simulink model "gm_HDLHeaderFull_vs"  (R2024a)
settings: Solver=FixedStepDiscrete  StartTime=0.0  StopTime=stopTime  RelTol=1e-3
values from neighbouring files (symbols this model uses):
  fs = 1    [testHeaderFull.m]
undefined symbols (not defined in the file or in its folder): clk, clk_enable, headerBitsPerFec, headerBitsPerOFDMSymbol, reset_x
libraries: hdlsllib x30, whdlutilities x6, simulink x5, dspsrcs4 x5, commhdlcrc x1, whdledac x1, vivadosimlib x1, HDL_ieee_8021513 x1
settings Model: Creator=cotti  LastModifiedBy=cotti
settings OptimizationCC: BlockReduction=off  ConditionallyExecuteInputs=off  DefaultParameterBehavior=Inlined  InheritOutputTypeSmallerThanSingle=on
settings DebuggingCC: AlgebraicLoopMsg=error  ArtificialAlgebraicLoopMsg=error  InheritedTsInSrcMsg=none  SingleTaskRateTransMsg=error  UnconnectedInputMsg=warning  UnconnectedOutputMsg=warning  UnconnectedLineMsg=warning
settings HardwareCC: ProdBitPerPointer=32  ProdBitPerSizeT=32  ProdBitPerPtrDiffT=32  ProdLargestAtomicFloat=None  ProdIntDivRoundTo=Undefined  ProdEndianess=Unspecified  ProdWordSize=32  ProdHWDeviceType=ASIC/FPGA->ASIC/FPGA  TargetBitPerLong=64  TargetBitPerPointer=64  TargetBitPerSizeT=64  TargetBitPerPtrDiffT=64  TargetLongLongMode=on  TargetIntDivRoundTo=Zero  TargetEndianess=LittleEndian  TargetWordSize=64  TargetHWDeviceType=Custom Processor->MATLAB Host Computer  ProdEqTarget=off

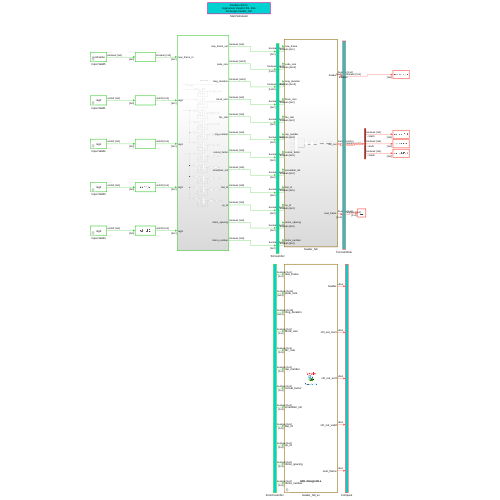
[thumbnail: Simulink's stored preview of the top-level diagram]
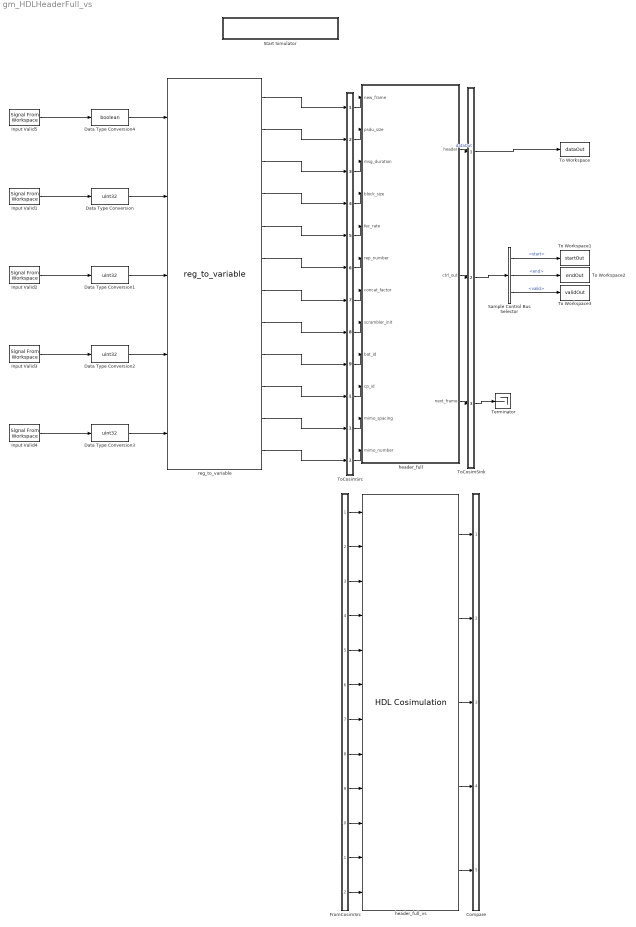
== system gm_HDLHeaderFull_vs ==
  Compare : Subsystem
      mask Display: disp('')
  Data Type Conversion{,1..3} (4 alike) : DataTypeConversion  OutDataTypeStr=uint32  SaturateOnIntegerOverflow=off  RndMeth=Floor
  Data Type Conversion4 : DataTypeConversion  OutDataTypeStr=boolean  SaturateOnIntegerOverflow=off  RndMeth=Floor
  FromCosimSrc : Subsystem
      mask Display: disp('')
  Input Valid1 : dspsrcs4/Signal From Workspace  X=reg0  Ts=1/fs  nsamps=1  OutputAfterFinalValue=Setting to zero  ignoreOrWarnInputAndFrameLengths=off  OutputFrames=off
  Input Valid2 : dspsrcs4/Signal From Workspace  X=reg1  Ts=1/fs  nsamps=1  OutputAfterFinalValue=Setting to zero  ignoreOrWarnInputAndFrameLengths=off  OutputFrames=off
  Input Valid3 : dspsrcs4/Signal From Workspace  X=reg2  Ts=1/fs  nsamps=1  OutputAfterFinalValue=Setting to zero  ignoreOrWarnInputAndFrameLengths=off  OutputFrames=off
  Input Valid4 : dspsrcs4/Signal From Workspace  X=reg3  Ts=1/fs  nsamps=1  OutputAfterFinalValue=Setting to zero  ignoreOrWarnInputAndFrameLengths=off  OutputFrames=off
  Input Valid5 : dspsrcs4/Signal From Workspace  X=newFrame  Ts=1/fs  nsamps=1  OutputAfterFinalValue=Setting to zero  ignoreOrWarnInputAndFrameLengths=off  OutputFrames=off
  Sample Control Bus Selector : whdlutilities/Sample Control Bus Selector  OutputSignals=start,end,valid
  Start Simulator : Subsystem
      settings: OpenFcn=|
      | cosimDirName = pwd;
      | cd 'hdl_prj_header_full/hdlsrc/HDLHeaderFull';
      | [s,r] = system('vivado -mode batch -source gm_HDLHeaderFull_vs.tcl','-echo');
      | cd (cosimDirName);
      | clear cosimDirName;
      | if s
      |    error('Failed to create Vivado HDL design DLL using script gm_HDLHeaderFull_vs.tcl.');
      | end
      mask Display: disp('Double-click to\nregenerate Vivado HDL DLL\nfor design header_full')
  Terminator : Terminator
  To Workspace : ToWorkspace  VariableName=dataOut  SampleTime=1/(8*fs)
      settings: Save2DSignal=2-D array (concatenate along first dimension)
  To Workspace1 : ToWorkspace  VariableName=startOut  SampleTime=1/(8*fs)
      settings: Save2DSignal=2-D array (concatenate along first dimension)
  To Workspace2 : ToWorkspace  VariableName=endOut  SampleTime=1/(8*fs)
      settings: Save2DSignal=2-D array (concatenate along first dimension)
  To Workspace3 : ToWorkspace  VariableName=validOut  SampleTime=1/(8*fs)
      settings: Save2DSignal=2-D array (concatenate along first dimension)
  ToCosimSink : Subsystem
      mask Display: disp('')
  ToCosimSrc : Subsystem
      mask Display: disp('')
  header_full : Subsystem
  header_full_vs : vivadosimlib/HDL Cosimulation  PortPaths=/header_full/new_frame;/header_full/psdu_size;/header_full/msg_duration;/header_full/block_size;/header_full/fec_rate;/header_full/rep_number;/header_full/concat_factor;/header_full/scrambler_init;/header_full/bat_id;/header_full/cp_id;/header_full/mimo_spacing;/header_full/mimo_number;/header_full/header;/header_full/ctrl_out_start;/header_full/ctrl_out_end;/header_full/ctrl_out_valid;/header_full/next_frame  PortModes=[1 1 1 1 1 1 1 1 1 1 1 1 2 2 2 2 2 ]  PortTimes=[-1 -1 -1 -1 -1 -1 -1 -1 -1 -1 -1 -1 0.125 0.125 0.125 0.125 0.125 ]  PortSigns=[-1 -1 -1 -1 -1 -1 -1 -1 -1 -1 -1 -1 0 0 0 0 0 ]  PortFracLengths=[0,0,0,0,0,0,0,0,0,0,0,0,0,0,0,0,0]  PortWordLengths=[-1,-1,-1,-1,-1,-1,-1,-1,-1,-1,-1,-1,1,1,1,1,1]  PortHDLWordSizes=[1,1,1,1,1,1,1,1,1,1,1,1,1,1,1,1,1]  CommLocal=on  CommSharedMemory=on  CommPortNumber=4449  CommShowInfo=on  ClockPaths=clk;clk_enable;reset_x;  ClockModes=[2 4 3]  ClockTimes=[1e-08 3.7e-08 2.7e-08]  TclPostSimCommand="puts \"done\""  TimingMode=ns  TimingScaleFactor=80  idxCellArray={'UNUSED_VAR'}  CosimBypass=Full Simulation  AllowDirectFeedthrough=on  ProductName=EDA Simulator Link VS  RunAutoTimescale=off  HdlClocks=0  PreRunTime=40  PreRunTimeUnit=ns
  reg_to_variable : HDL_ieee_8021513/reg_to_variable  SystemSampleTime=-1  VariantActivationTime=update diagram  AllowFlexibleInterface=on  Latency=0  AutoFrameSizeCalculation=off
      settings: SourceProductName=HDL IEEE 8021513
  wires:
  Sample Control Bus Selector/2 -> To Workspace2/1  "<end>"
  Sample Control Bus Selector/3 -> To Workspace3/1  "<valid>"
  Sample Control Bus Selector/1 -> To Workspace1/1  "<start>"
  Data Type Conversion/1 -> reg_to_variable/2
  Data Type Conversion1/1 -> reg_to_variable/3
  Data Type Conversion2/1 -> reg_to_variable/4
  Data Type Conversion3/1 -> reg_to_variable/5
  Data Type Conversion4/1 -> reg_to_variable/1
  Input Valid4/1 -> Data Type Conversion3/1
  Input Valid3/1 -> Data Type Conversion2/1
  Input Valid2/1 -> Data Type Conversion1/1
  Input Valid1/1 -> Data Type Conversion/1
  Input Valid5/1 -> Data Type Conversion4/1
  ToCosimSrc/1(out1) -> header_full/1(new_frame)
  ToCosimSrc/2(out2) -> header_full/2(psdu_size)
  ToCosimSrc/3(out3) -> header_full/3(msg_duration)
  ToCosimSrc/4(out4) -> header_full/4(block_size)
  ToCosimSrc/5(out5) -> header_full/5(fec_rate)
  ToCosimSrc/6(out6) -> header_full/6(rep_number)
  ToCosimSrc/7(out7) -> header_full/7(concat_factor)
  ToCosimSrc/8(out8) -> header_full/8(scrambler_init)
  ToCosimSrc/9(out9) -> header_full/9(bat_id)
  ToCosimSrc/10(out10) -> header_full/10(cp_id)
  ToCosimSrc/11(out11) -> header_full/11(mimo_spacing)
  ToCosimSrc/12(out12) -> header_full/12(mimo_number)
  header_full/1(header) -> ToCosimSink/1(in1)  "dataOut"
  header_full/2(ctrl_out) -> ToCosimSink/2(in2)
  header_full/3(next_frame) -> ToCosimSink/3(in3)
  reg_to_variable/1 -> ToCosimSrc/1(in1)
  reg_to_variable/2 -> ToCosimSrc/2(in2)
  reg_to_variable/3 -> ToCosimSrc/3(in3)
  reg_to_variable/4 -> ToCosimSrc/4(in4)
  reg_to_variable/5 -> ToCosimSrc/5(in5)
  reg_to_variable/6 -> ToCosimSrc/6(in6)
  reg_to_variable/7 -> ToCosimSrc/7(in7)
  reg_to_variable/8 -> ToCosimSrc/8(in8)
  reg_to_variable/9 -> ToCosimSrc/9(in9)
  reg_to_variable/10 -> ToCosimSrc/10(in10)
  reg_to_variable/11 -> ToCosimSrc/11(in11)
  reg_to_variable/12 -> ToCosimSrc/12(in12)
  ToCosimSink/1(out1) -> To Workspace/1
  ToCosimSink/2(out2) -> Sample Control Bus Selector/1
  ToCosimSink/3(out3) -> Terminator/1
  FromCosimSrc/1(out1) -> header_full_vs/1
  FromCosimSrc/2(out2) -> header_full_vs/2
  FromCosimSrc/3(out3) -> header_full_vs/3
  FromCosimSrc/4(out4) -> header_full_vs/4
  FromCosimSrc/5(out5) -> header_full_vs/5
  FromCosimSrc/6(out6) -> header_full_vs/6
  FromCosimSrc/7(out7) -> header_full_vs/7
  FromCosimSrc/8(out8) -> header_full_vs/8
  FromCosimSrc/9(out9) -> header_full_vs/9
  FromCosimSrc/10(out10) -> header_full_vs/10
  FromCosimSrc/11(out11) -> header_full_vs/11
  FromCosimSrc/12(out12) -> header_full_vs/12
  header_full_vs/1 -> Compare/1(in1)
  header_full_vs/2 -> Compare/2(in2)
  header_full_vs/3 -> Compare/3(in3)
  header_full_vs/4 -> Compare/4(in4)
  header_full_vs/5 -> Compare/5(in5)

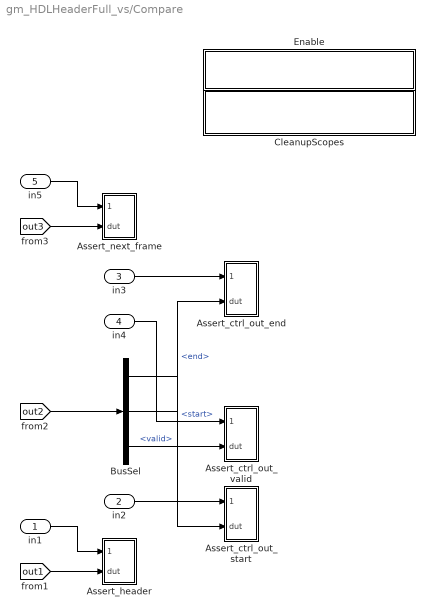
== system gm_HDLHeaderFull_vs/Compare ==
  in1 : Inport
  in2 : Inport  Port=2
  in3 : Inport  Port=3
  in4 : Inport  Port=4
  in5 : Inport  Port=5
  Assert_ctrl_out_end : Subsystem
      settings: LibrarySourceBlock=hdlmdlgenlib/AssertEq
  Assert_ctrl_out_start : Subsystem
      settings: LibrarySourceBlock=hdlmdlgenlib/AssertEq
  Assert_ctrl_out_valid : Subsystem
      settings: LibrarySourceBlock=hdlmdlgenlib/AssertEq
  Assert_header : Subsystem
      settings: LibrarySourceBlock=hdlmdlgenlib/AssertEq
  Assert_next_frame : Subsystem
      settings: LibrarySourceBlock=hdlmdlgenlib/AssertEq
  BusSel : BusSelector  OutputSignals=start,end,valid
  CleanupScopes : Subsystem
      settings: OpenFcn=|
      | blkName = gcb; %self block
      | idx = regexp(blkName, '/CleanupScopes$', 'once');
      | blkParent = blkName(1:idx-1);
      | blks=find_system(blkParent, 'LookUnderMasks', 'all','blocktype', 'Scope');
      | for itr = 1:length(blks)
      | 	 hScopeCfg = get_param(blks{itr},'ScopeConfiguration');
      | 	 hScopeCfg.Visible = ~ hScopeCfg.Visible;
      | end
      | drawnow;
      mask Display: fprintf(message('hdlcoder:cosim:vnl_dblclick').getString());
  Enable : Subsystem
      settings: OpenFcn=|
      | blkName = gcb;
      | idx = regexp(blkName, '/Enable$', 'once');
      | blkParent = blkName(1:idx-1);
      | blks=find_system(blkParent, 'LookUnderMasks', 'all','blocktype', 'Assertion');
      | e = get_param(blks{1}, 'Enabled');
      | if strcmp(e, 'on'), f= 'off';, else, f = 'on';, end
      | for ii=1:length(blks), set_param(blks{ii}, 'Enabled', f);, end
      | set_param(gcb, 'MaskDisplay',['fprintf(message(''hdlcoder:cosim:vnl_dblclick_assertions'',','''',upper(e),'''',').getString())']);
      mask Display: fprintf(message('hdlcoder:cosim:vnl_dblclick_assertions','OFF').getString());
  wires:
  in2/1 -> Assert_ctrl_out_start/1(cosim)
  BusSel/1 -> Assert_ctrl_out_start/2(dut)  "<start>"
  in3/1 -> Assert_ctrl_out_end/1(cosim)
  BusSel/3 -> Assert_ctrl_out_valid/2(dut)  "<valid>"
  [out1] -> Assert_header/2(dut)
  in1/1 -> Assert_header/1(cosim)
  BusSel/2 -> Assert_ctrl_out_end/2(dut)  "<end>"
  in4/1 -> Assert_ctrl_out_valid/1(cosim)
  [out2] -> BusSel/1
  [out3] -> Assert_next_frame/2(dut)
  in5/1 -> Assert_next_frame/1(cosim)

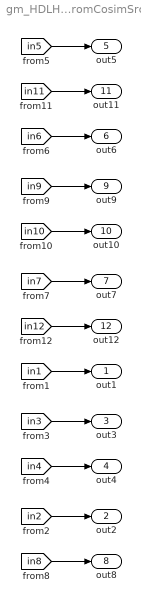
== system gm_HDLHeaderFull_vs/FromCosimSrc ==
  out1 : Outport
  out2 : Outport  Port=2
  out3 : Outport  Port=3
  out4 : Outport  Port=4
  out5 : Outport  Port=5
  out6 : Outport  Port=6
  out7 : Outport  Port=7
  out8 : Outport  Port=8
  out9 : Outport  Port=9
  out10 : Outport  Port=10
  out11 : Outport  Port=11
  out12 : Outport  Port=12
  wires:
  [in8] -> out8/1
  [in2] -> out2/1
  [in4] -> out4/1
  [in3] -> out3/1
  [in7] -> out7/1
  [in10] -> out10/1
  [in9] -> out9/1
  [in12] -> out12/1
  [in6] -> out6/1
  [in1] -> out1/1
  [in11] -> out11/1
  [in5] -> out5/1

== system gm_HDLHeaderFull_vs/Start Simulator ==

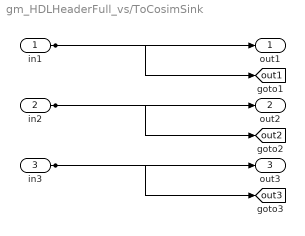
== system gm_HDLHeaderFull_vs/ToCosimSink ==
  in1 : Inport
  in2 : Inport  Port=2
  in3 : Inport  Port=3
  out1 : Outport
  out2 : Outport  Port=2
  out3 : Outport  Port=3
  tag scope: out1=global, out2=global, out3=global
  wires:
  in1/1 -> out1/1, [out1]
  in2/1 -> out2/1, [out2]
  in3/1 -> out3/1, [out3]

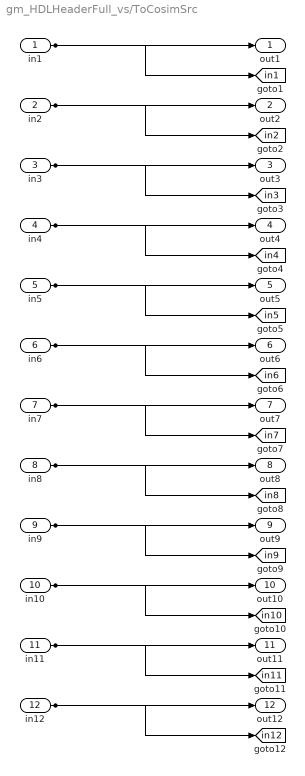
== system gm_HDLHeaderFull_vs/ToCosimSrc ==
  in1 : Inport
  in2 : Inport  Port=2
  in3 : Inport  Port=3
  in4 : Inport  Port=4
  in5 : Inport  Port=5
  in6 : Inport  Port=6
  in7 : Inport  Port=7
  in8 : Inport  Port=8
  in9 : Inport  Port=9
  in10 : Inport  Port=10
  in11 : Inport  Port=11
  in12 : Inport  Port=12
  out1 : Outport
  out2 : Outport  Port=2
  out3 : Outport  Port=3
  out4 : Outport  Port=4
  out5 : Outport  Port=5
  out6 : Outport  Port=6
  out7 : Outport  Port=7
  out8 : Outport  Port=8
  out9 : Outport  Port=9
  out10 : Outport  Port=10
  out11 : Outport  Port=11
  out12 : Outport  Port=12
  tag scope: in10=global, in11=global, in12=global, in1=global, in2=global, in3=global, in4=global, in5=global, in6=global, in7=global, in8=global, in9=global
  wires:
  in1/1 -> out1/1, [in1]
  in2/1 -> out2/1, [in2]
  in3/1 -> out3/1, [in3]
  in4/1 -> out4/1, [in4]
  in5/1 -> out5/1, [in5]
  in6/1 -> out6/1, [in6]
  in7/1 -> out7/1, [in7]
  in8/1 -> out8/1, [in8]
  in9/1 -> out9/1, [in9]
  in10/1 -> out10/1, [in10]
  in11/1 -> out11/1, [in11]
  in12/1 -> out12/1, [in12]

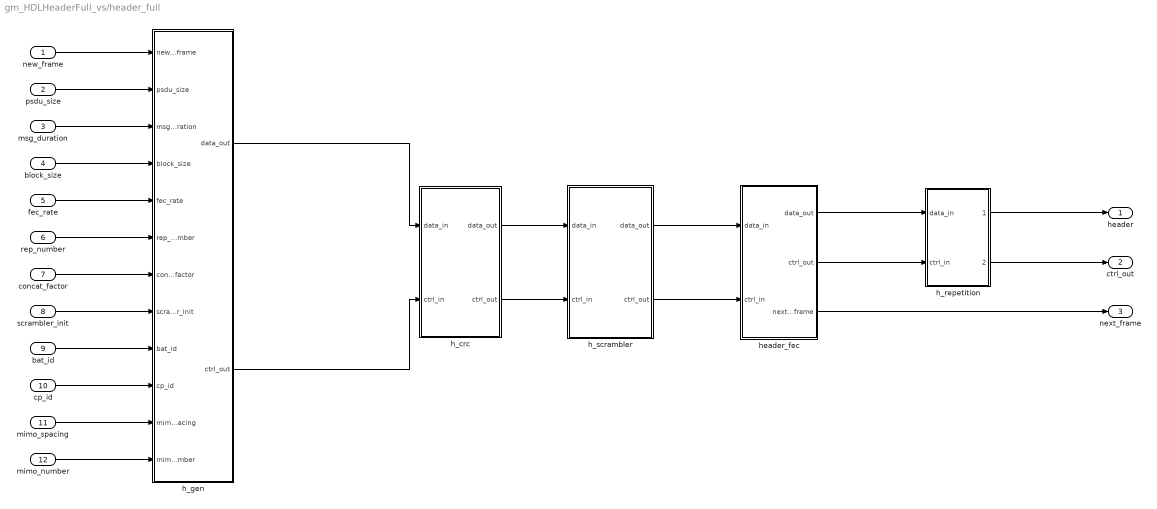
== system gm_HDLHeaderFull_vs/header_full ==
  new_frame : Inport  OutDataTypeStr=boolean  SampleTime=1
  psdu_size : Inport  Port=2  OutDataTypeStr=boolean  PortDimensions=[1 24]  SampleTime=1
  msg_duration : Inport  Port=3  OutDataTypeStr=boolean  PortDimensions=[1 16]  SampleTime=1
  block_size : Inport  Port=4  OutDataTypeStr=boolean  PortDimensions=[1 2]  SampleTime=1
  fec_rate : Inport  Port=5  OutDataTypeStr=boolean  PortDimensions=[1 3]  SampleTime=1
  rep_number : Inport  Port=6  OutDataTypeStr=boolean  PortDimensions=[1 3]  SampleTime=1
  concat_factor : Inport  Port=7  OutDataTypeStr=boolean  PortDimensions=[1 3]  SampleTime=1
  scrambler_init : Inport  Port=8  OutDataTypeStr=boolean  PortDimensions=[1 4]  SampleTime=1
  bat_id : Inport  Port=9  OutDataTypeStr=boolean  PortDimensions=[1 5]  SampleTime=1
  cp_id : Inport  Port=10  OutDataTypeStr=boolean  PortDimensions=[1 3]  SampleTime=1
  mimo_spacing : Inport  Port=11  OutDataTypeStr=boolean  PortDimensions=[1 3]  SampleTime=1
  mimo_number : Inport  Port=12  OutDataTypeStr=boolean  PortDimensions=[1 3]  SampleTime=1
  h_crc : Subsystem
  h_gen : Subsystem
  h_repetition : Subsystem
  h_scrambler : Subsystem
  header_fec : Subsystem
  header : Outport  SampleTime=0.125
  ctrl_out : Outport  Port=2  SampleTime=0.125
  next_frame : Outport  Port=3  SampleTime=0.125
  wires:
  header_fec/3(next_frame) -> next_frame/1
  header_fec/2(ctrl_out) -> h_repetition/2(ctrl_in)
  header_fec/1(data_out) -> h_repetition/1(data_in)
  h_scrambler/2(ctrl_out) -> header_fec/2(ctrl_in)
  h_scrambler/1(data_out) -> header_fec/1(data_in)
  h_repetition/2(ctrl_out) -> ctrl_out/1
  h_repetition/1(data_out) -> header/1
  h_gen/2(ctrl_out) -> h_crc/2(ctrl_in)
  h_gen/1(data_out) -> h_crc/1(data_in)
  h_crc/2(ctrl_out) -> h_scrambler/2(ctrl_in)
  h_crc/1(data_out) -> h_scrambler/1(data_in)
  mimo_number/1 -> h_gen/12(mimo_number)
  mimo_spacing/1 -> h_gen/11(mimo_spacing)
  cp_id/1 -> h_gen/10(cp_id)
  bat_id/1 -> h_gen/9(bat_id)
  scrambler_init/1 -> h_gen/8(scrambler_init)
  concat_factor/1 -> h_gen/7(concat_factor)
  rep_number/1 -> h_gen/6(rep_number)
  fec_rate/1 -> h_gen/5(fec_rate)
  block_size/1 -> h_gen/4(block_size)
  msg_duration/1 -> h_gen/3(msg_duration)
  psdu_size/1 -> h_gen/2(psdu_size)
  new_frame/1 -> h_gen/1(new_frame)

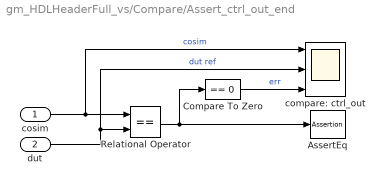
== system gm_HDLHeaderFull_vs/Compare/Assert_ctrl_out_end ==
  cosim : Inport
  dut : Inport  Port=2
  AssertEq : Assertion
  Compare To Zero : simulink/Logic and Bit Operations/Compare To Zero  relop===  OutDataTypeStr=boolean
  Relational Operator : RelationalOperator  Operator===  OutDataTypeStr=boolean  InputSameDT=off
  compare: ctrl_out : Scope  NumInputPorts=3
  wires:
  Compare To Zero/1 -> compare: ctrl_out/3  "err"
  Relational Operator/1 -> Compare To Zero/1, AssertEq/1
  cosim/1 -> compare: ctrl_out/1, Relational Operator/1  "cosim"
  dut/1 -> compare: ctrl_out/2, Relational Operator/2  "dut ref"

== system gm_HDLHeaderFull_vs/Compare/Assert_ctrl_out_start ==
  cosim : Inport
  dut : Inport  Port=2
  AssertEq : Assertion
  Compare To Zero : simulink/Logic and Bit Operations/Compare To Zero  relop===  OutDataTypeStr=boolean
  Relational Operator : RelationalOperator  Operator===  OutDataTypeStr=boolean  InputSameDT=off
  compare: ctrl_out : Scope  NumInputPorts=3
  wires:
  Compare To Zero/1 -> compare: ctrl_out/3  "err"
  Relational Operator/1 -> Compare To Zero/1, AssertEq/1
  cosim/1 -> compare: ctrl_out/1, Relational Operator/1  "cosim"
  dut/1 -> compare: ctrl_out/2, Relational Operator/2  "dut ref"

== system gm_HDLHeaderFull_vs/Compare/Assert_ctrl_out_valid ==
  cosim : Inport
  dut : Inport  Port=2
  AssertEq : Assertion
  Compare To Zero : simulink/Logic and Bit Operations/Compare To Zero  relop===  OutDataTypeStr=boolean
  Relational Operator : RelationalOperator  Operator===  OutDataTypeStr=boolean  InputSameDT=off
  compare: ctrl_out : Scope  NumInputPorts=3
  wires:
  Compare To Zero/1 -> compare: ctrl_out/3  "err"
  Relational Operator/1 -> Compare To Zero/1, AssertEq/1
  cosim/1 -> compare: ctrl_out/1, Relational Operator/1  "cosim"
  dut/1 -> compare: ctrl_out/2, Relational Operator/2  "dut ref"

== system gm_HDLHeaderFull_vs/Compare/Assert_header ==
  cosim : Inport
  dut : Inport  Port=2
  AssertEq : Assertion
  Compare To Zero : simulink/Logic and Bit Operations/Compare To Zero  relop===  OutDataTypeStr=boolean
  Relational Operator : RelationalOperator  Operator===  OutDataTypeStr=boolean  InputSameDT=off
  compare: header : Scope  NumInputPorts=3
  wires:
  Compare To Zero/1 -> compare: header/3  "err"
  Relational Operator/1 -> Compare To Zero/1, AssertEq/1
  cosim/1 -> compare: header/1, Relational Operator/1  "cosim"
  dut/1 -> compare: header/2, Relational Operator/2  "dut ref"

== system gm_HDLHeaderFull_vs/Compare/Assert_next_frame ==
  cosim : Inport
  dut : Inport  Port=2
  AssertEq : Assertion
  Compare To Zero : simulink/Logic and Bit Operations/Compare To Zero  relop===  OutDataTypeStr=boolean
  Relational Operator : RelationalOperator  Operator===  OutDataTypeStr=boolean  InputSameDT=off
  compare: next_frame : Scope  NumInputPorts=3
  wires:
  Compare To Zero/1 -> compare: next_frame/3  "err"
  Relational Operator/1 -> Compare To Zero/1, AssertEq/1
  cosim/1 -> compare: next_frame/1, Relational Operator/1  "cosim"
  dut/1 -> compare: next_frame/2, Relational Operator/2  "dut ref"

== system gm_HDLHeaderFull_vs/Compare/CleanupScopes ==

== system gm_HDLHeaderFull_vs/Compare/Enable ==

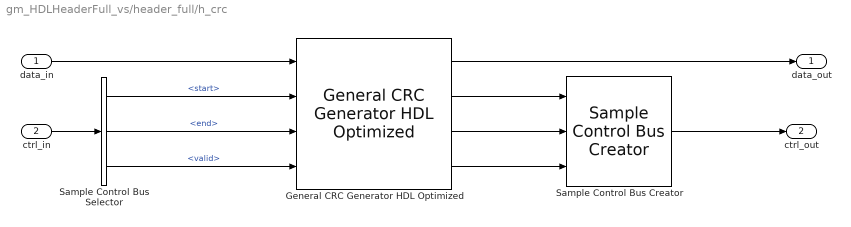
== system gm_HDLHeaderFull_vs/header_full/h_crc ==
  data_in : Inport  OutDataTypeStr=boolean  SampleTime=0.125
  ctrl_in : Inport  Port=2  SampleTime=0.125
  General CRC Generator HDL Optimized : commhdlcrc/General CRC Generator HDL Optimized  Polynomial=headerCRCPoly  InitialState=1  DirectMethod=on  ReflectInput=off  ReflectCRCChecksum=off  FinalXORValue=0  SimulateUsing=Code generation
  Sample Control Bus Creator : whdlutilities/Sample Control Bus Creator
  Sample Control Bus Selector : whdlutilities/Sample Control Bus Selector  OutputSignals=start,end,valid
  data_out : Outport  SampleTime=0.125
  ctrl_out : Outport  Port=2  SampleTime=0.125
  wires:
  Sample Control Bus Selector/3 -> General CRC Generator HDL Optimized/4  "<valid>"
  Sample Control Bus Selector/2 -> General CRC Generator HDL Optimized/3  "<end>"
  Sample Control Bus Selector/1 -> General CRC Generator HDL Optimized/2  "<start>"
  Sample Control Bus Creator/1 -> ctrl_out/1
  General CRC Generator HDL Optimized/4 -> Sample Control Bus Creator/3
  General CRC Generator HDL Optimized/3 -> Sample Control Bus Creator/2
  General CRC Generator HDL Optimized/2 -> Sample Control Bus Creator/1
  General CRC Generator HDL Optimized/1 -> data_out/1
  ctrl_in/1 -> Sample Control Bus Selector/1
  data_in/1 -> General CRC Generator HDL Optimized/1

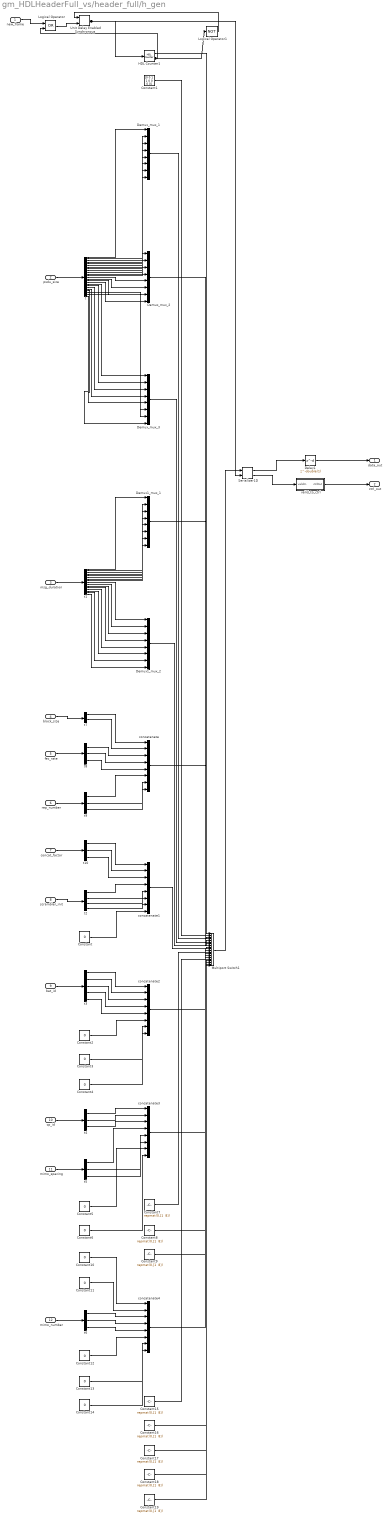
== system gm_HDLHeaderFull_vs/header_full/h_gen ==
  new_frame : Inport  OutDataTypeStr=boolean  SampleTime=1
  psdu_size : Inport  Port=2  OutDataTypeStr=boolean  PortDimensions=[1 24]  SampleTime=1
  msg_duration : Inport  Port=3  OutDataTypeStr=boolean  PortDimensions=[1 16]  SampleTime=1
  block_size : Inport  Port=4  OutDataTypeStr=boolean  PortDimensions=[1 2]  SampleTime=1
  fec_rate : Inport  Port=5  OutDataTypeStr=boolean  PortDimensions=[1 3]  SampleTime=1
  rep_number : Inport  Port=6  OutDataTypeStr=boolean  PortDimensions=[1 3]  SampleTime=1
  concat_factor : Inport  Port=7  OutDataTypeStr=boolean  PortDimensions=[1 3]  SampleTime=1
  scrambler_init : Inport  Port=8  OutDataTypeStr=boolean  PortDimensions=[1 4]  SampleTime=1
  bat_id : Inport  Port=9  OutDataTypeStr=boolean  PortDimensions=[1 5]  SampleTime=1
  cp_id : Inport  Port=10  OutDataTypeStr=boolean  PortDimensions=[1 3]  SampleTime=1
  mimo_spacing : Inport  Port=11  OutDataTypeStr=boolean  PortDimensions=[1 3]  SampleTime=1
  mimo_number : Inport  Port=12  OutDataTypeStr=boolean  PortDimensions=[1 3]  SampleTime=1
  Constant{,2..6,10..14} (11 alike) : Constant  Value=0  OutDataTypeStr=boolean  SampleTime=1
  Constant1 : Constant  Value=[0 0 1 1 0 0 0 0]  VectorParams1D=off  OutDataTypeStr=boolean  SampleTime=1
  Constant{7..9,15..19} (8 alike) : Constant  Value="repmat(0,[1  8])"  VectorParams1D=off  OutDataTypeStr=boolean  SampleTime=1
  Delay1 : Delay  DelayLength=double(1)  InitialCondition=0  SampleTime=0.125
  Demux1_mux_1 : Mux  Inputs=8
  Demux1_mux_2 : Mux  Inputs=8
  Demux_mux_1 : Mux  Inputs=8
  Demux_mux_2 : Mux  Inputs=8
  Demux_mux_3 : Mux  Inputs=8
  HDL Counter1 : hdlsllib/Sources/HDL Counter  CountType=Count limited  CountInit=0  CountStep=1  CountMax=18  CountFromType=Initial value  CountFrom=0  CountResetPort=off  CountLoadPort=off  CountEnbPort=on  CountDirPort=off  CountHitOutputPort=on  CountDataType=Unsigned  CountWordLen=5  CountFracLen=0  CountSampTime=1
  Logical Operator : Logic  Operator=OR  AllPortsSameDT=off  OutDataTypeStr=boolean  SampleTime=1
  Logical Operator1 : Logic  Operator=NOT  Inputs=1  AllPortsSameDT=off  OutDataTypeStr=boolean  SampleTime=1
  Multiport Switch1 : MultiPortSwitch  DataPortOrder=Zero-based contiguous  Inputs=19  DiagnosticForDefault=None  zeroidx=on  SampleTime=1  SaturateOnIntegerOverflow=off  InputSameDT=off
  Serializer1D : hdlsllib/HDL Operations/Serializer1D  Ratio=8  IdleCycles=0  validIn=on  startOut=off  validOut=on  inputDataDimensions=8  inputSampleTime=1  inputSignalType=real
  Unit Delay Enabled Synchronous : hdlsllib/Discrete/Unit Delay Enabled Synchronous  InitialCondition=double(0)  SampleTime=-1
  concatenate{,1..4} (5 alike) : Concatenate  NumInputs=8  Mode=Multidimensional array  ConcatenateDimension=2
  t : Demux  Outputs=24
  t1 : Demux  Outputs=16
  t{4..6,8..10} (6 alike) : Demux  Outputs=3
  t2 : Demux
  t3 : Demux  Outputs=5
  t7 : Demux  Outputs=2
  valid_to_ctrl : Subsystem
  data_out : Outport  SampleTime=0.125
  ctrl_out : Outport  Port=2  SampleTime=0.125
  wires:
  t10/3 -> concatenate1/3
  t10/2 -> concatenate1/2
  t10/1 -> concatenate1/1
  t9/3 -> concatenate/8
  t9/2 -> concatenate/7
  t9/1 -> concatenate/6
  t8/3 -> concatenate/5
  t8/2 -> concatenate/4
  t8/1 -> concatenate/3
  t7/2 -> concatenate/2
  t7/1 -> concatenate/1
  t6/3 -> concatenate4/5
  t6/2 -> concatenate4/4
  t6/1 -> concatenate4/3
  t5/3 -> concatenate3/6
  t5/2 -> concatenate3/5
  t5/1 -> concatenate3/4
  t4/3 -> concatenate3/3
  t4/2 -> concatenate3/2
  t4/1 -> concatenate3/1
  t3/5 -> concatenate2/5
  t3/4 -> concatenate2/4
  t3/3 -> concatenate2/3
  t3/2 -> concatenate2/2
  t3/1 -> concatenate2/1
  t2/4 -> concatenate1/7
  t2/3 -> concatenate1/6
  t2/2 -> concatenate1/5
  t2/1 -> concatenate1/4
  t1/16 -> Demux1_mux_2/8
  t1/15 -> Demux1_mux_2/7
  t1/14 -> Demux1_mux_2/6
  t1/13 -> Demux1_mux_2/5
  t1/12 -> Demux1_mux_2/4
  t1/11 -> Demux1_mux_2/3
  t1/10 -> Demux1_mux_2/2
  t1/9 -> Demux1_mux_2/1
  t1/8 -> Demux1_mux_1/8
  t1/7 -> Demux1_mux_1/7
  t1/6 -> Demux1_mux_1/6
  t1/5 -> Demux1_mux_1/5
  t1/4 -> Demux1_mux_1/4
  t1/3 -> Demux1_mux_1/3
  t1/2 -> Demux1_mux_1/2
  t1/1 -> Demux1_mux_1/1
  t/24 -> Demux_mux_3/8
  t/23 -> Demux_mux_3/7
  t/22 -> Demux_mux_3/6
  t/21 -> Demux_mux_3/5
  t/20 -> Demux_mux_3/4
  t/19 -> Demux_mux_3/3
  t/18 -> Demux_mux_3/2
  t/17 -> Demux_mux_3/1
  t/16 -> Demux_mux_2/8
  t/15 -> Demux_mux_2/7
  t/14 -> Demux_mux_2/6
  t/13 -> Demux_mux_2/5
  t/12 -> Demux_mux_2/4
  t/11 -> Demux_mux_2/3
  t/10 -> Demux_mux_2/2
  t/9 -> Demux_mux_2/1
  t/8 -> Demux_mux_1/8
  t/7 -> Demux_mux_1/7
  t/6 -> Demux_mux_1/6
  t/5 -> Demux_mux_1/5
  t/4 -> Demux_mux_1/4
  t/3 -> Demux_mux_1/3
  t/2 -> Demux_mux_1/2
  t/1 -> Demux_mux_1/1
  valid_to_ctrl/1(ctrlOut) -> ctrl_out/1
  concatenate4/1 -> Multiport Switch1/15
  concatenate3/1 -> Multiport Switch1/11
  concatenate2/1 -> Multiport Switch1/10
  concatenate1/1 -> Multiport Switch1/9
  concatenate/1 -> Multiport Switch1/8
  Unit Delay Enabled Synchronous/1 -> HDL Counter1/1, Serializer1D/2
  Serializer1D/2 -> valid_to_ctrl/1(validIn)
  Serializer1D/1 -> Delay1/1
  Multiport Switch1/1 -> Serializer1D/1
  Logical Operator1/1 -> Unit Delay Enabled Synchronous/1
  Logical Operator/1 -> Unit Delay Enabled Synchronous/2
  HDL Counter1/2 -> Logical Operator/2, Logical Operator1/1
  HDL Counter1/1 -> Multiport Switch1/1
  Demux1_mux_2/1 -> Multiport Switch1/7
  Demux1_mux_1/1 -> Multiport Switch1/6
  Demux_mux_3/1 -> Multiport Switch1/5
  Demux_mux_2/1 -> Multiport Switch1/4
  Demux_mux_1/1 -> Multiport Switch1/3
  Delay1/1 -> data_out/1
  Constant9/1 -> Multiport Switch1/14
  Constant8/1 -> Multiport Switch1/13
  Constant7/1 -> Multiport Switch1/12
  Constant6/1 -> concatenate3/8
  Constant5/1 -> concatenate3/7
  Constant4/1 -> concatenate2/8
  Constant3/1 -> concatenate2/7
  Constant2/1 -> concatenate2/6
  Constant19/1 -> Multiport Switch1/20
  Constant18/1 -> Multiport Switch1/19
  Constant17/1 -> Multiport Switch1/18
  Constant16/1 -> Multiport Switch1/17
  Constant15/1 -> Multiport Switch1/16
  Constant14/1 -> concatenate4/8
  Constant13/1 -> concatenate4/7
  Constant12/1 -> concatenate4/6
  Constant11/1 -> concatenate4/2
  Constant10/1 -> concatenate4/1
  Constant1/1 -> Multiport Switch1/2
  Constant/1 -> concatenate1/8
  mimo_number/1 -> t6/1
  mimo_spacing/1 -> t5/1
  cp_id/1 -> t4/1
  bat_id/1 -> t3/1
  scrambler_init/1 -> t2/1
  concat_factor/1 -> t10/1
  rep_number/1 -> t9/1
  fec_rate/1 -> t8/1
  block_size/1 -> t7/1
  msg_duration/1 -> t1/1
  psdu_size/1 -> t/1
  new_frame/1 -> Logical Operator/1

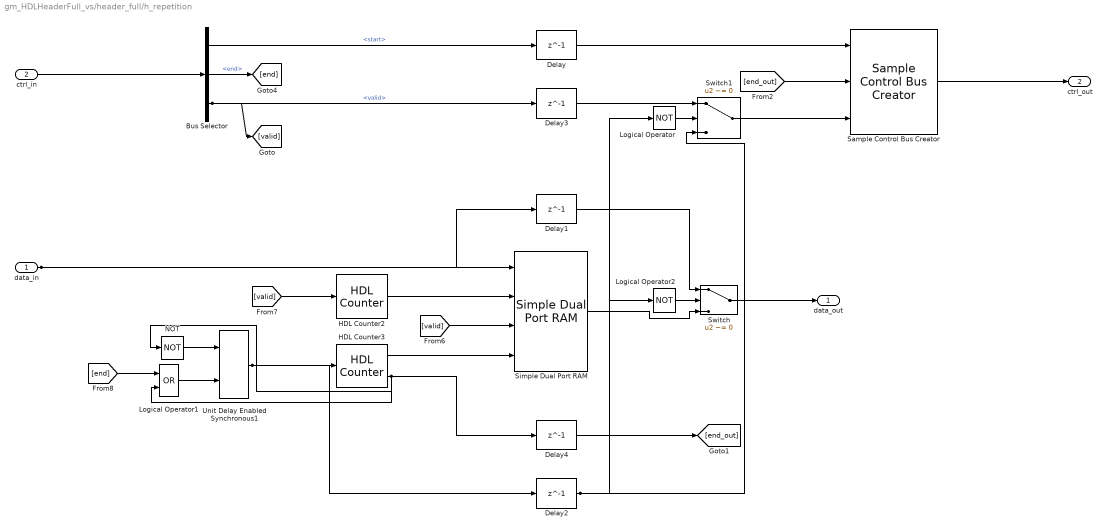
== system gm_HDLHeaderFull_vs/header_full/h_repetition ==
  data_in : Inport  OutDataTypeStr=boolean  SampleTime=0.125
  ctrl_in : Inport  Port=2  SampleTime=0.125
  Bus Selector : BusSelector  OutputSignals=start,end,valid
  Delay{,1..4} (5 alike) : Delay  DelayLength=1  InitialCondition=0  UseCircularBuffer=on
  HDL Counter2 : hdlsllib/Sources/HDL Counter  CountType=Count limited  CountInit=headerBitsPerFec-2  CountStep=1  CountMax=headerBitsPerFec-1  CountFromType=Specify  CountFrom=0  CountResetPort=off  CountLoadPort=off  CountEnbPort=on  CountDirPort=off  CountHitOutputPort=off  CountDataType=Unsigned  CountWordLen=nextpow2(headerBitsPerOFDMSymbol)  CountFracLen=0  CountSampTime=1
  HDL Counter3 : hdlsllib/Sources/HDL Counter  CountType=Count limited  CountInit=0  CountStep=1  CountMax=headerBitsPerOFDMSymbol - headerBitsPerFec -1  CountFromType=Initial value  CountFrom=0  CountResetPort=off  CountLoadPort=off  CountEnbPort=on  CountDirPort=off  CountHitOutputPort=on  CountDataType=Unsigned  CountWordLen=nextpow2(headerBitsPerOFDMSymbol)  CountFracLen=0  CountSampTime=1
  Logical Operator : Logic  Operator=NOT  IconShape=distinctive  AllPortsSameDT=off  OutDataTypeStr=boolean
  Logical Operator1 : Logic  Operator=OR  IconShape=distinctive  AllPortsSameDT=off  OutDataTypeStr=boolean
  Logical Operator2 : Logic  Operator=NOT  IconShape=distinctive  AllPortsSameDT=off  OutDataTypeStr=boolean
  NOT : Logic  Operator=NOT  IconShape=distinctive  AllPortsSameDT=off  OutDataTypeStr=boolean
  Sample Control Bus Creator : whdlutilities/Sample Control Bus Creator
  Simple Dual Port RAM : hdlsllib/HDL RAMs/Simple Dual Port RAM  ram_size=nextpow2(headerBitsPerOFDMSymbol)
  Switch : Switch  Criteria=u2 ~= 0  OutDataTypeStr=boolean  SaturateOnIntegerOverflow=off  InputSameDT=off
  Switch1 : Switch  Criteria=u2 ~= 0  OutDataTypeStr=boolean  SaturateOnIntegerOverflow=off  InputSameDT=off
  Unit Delay Enabled Synchronous1 : hdlsllib/Discrete/Unit Delay Enabled Synchronous  InitialCondition=0.0  SampleTime=-1
  data_out : Outport  SampleTime=0.125
  ctrl_out : Outport  Port=2  SampleTime=0.125
  wires:
  Unit Delay Enabled Synchronous1/1 -> HDL Counter3/1, Delay2/1
  Switch1/1 -> Sample Control Bus Creator/3
  Switch/1 -> data_out/1
  Simple Dual Port RAM/1 -> Switch/3
  Sample Control Bus Creator/1 -> ctrl_out/1
  NOT/1 -> Unit Delay Enabled Synchronous1/1
  Logical Operator2/1 -> Switch/2
  Logical Operator1/1 -> Unit Delay Enabled Synchronous1/2
  Logical Operator/1 -> Switch1/2
  HDL Counter3/2 -> Delay4/1, Logical Operator1/2, NOT/1
  HDL Counter3/1 -> Simple Dual Port RAM/4
  HDL Counter2/1 -> Simple Dual Port RAM/2
  [end] -> Logical Operator1/1
  [valid] -> HDL Counter2/1
  [valid] -> Simple Dual Port RAM/3
  [end_out] -> Sample Control Bus Creator/2
  Delay4/1 -> [end_out]
  Delay3/1 -> Switch1/1
  Delay2/1 -> Logical Operator/1, Logical Operator2/1, Switch1/3
  Delay1/1 -> Switch/1
  Delay/1 -> Sample Control Bus Creator/1
  Bus Selector/3 -> Delay3/1, [valid]  "<valid>"
  Bus Selector/2 -> [end]  "<end>"
  Bus Selector/1 -> Delay/1  "<start>"
  ctrl_in/1 -> Bus Selector/1
  data_in/1 -> Simple Dual Port RAM/1, Delay1/1

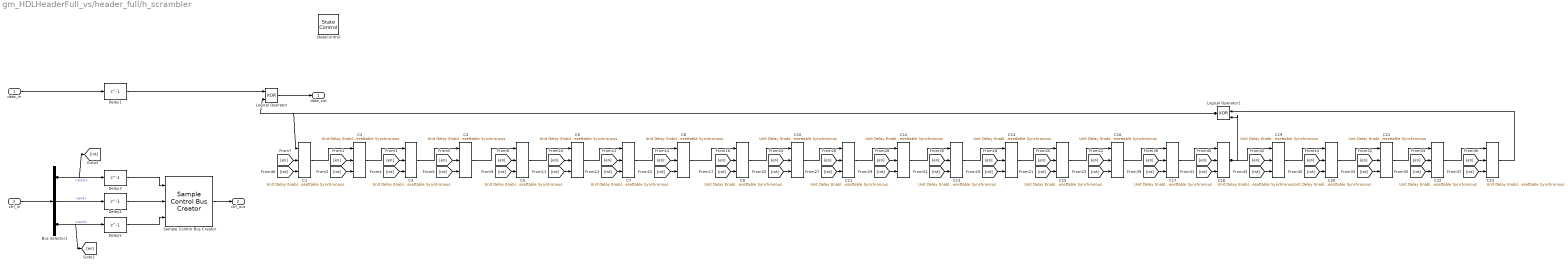
== system gm_HDLHeaderFull_vs/header_full/h_scrambler ==
  data_in : Inport  OutDataTypeStr=boolean  SampleTime=0.125
  ctrl_in : Inport  Port=2  SampleTime=0.125
  Bus Selector1 : BusSelector  OutputSignals=start,end,valid
  C{1,3,5,7,9,11,13,15,17,19,21,23} (12 alike) : hdlsllib/Discrete/Unit Delay Enabled Resettable Synchronous  InitialCondition=0  SampleTime=-1
  C{2,4,6,8,10,12,14,16,18,20,22} (11 alike) : hdlsllib/Discrete/Unit Delay Enabled Resettable Synchronous  InitialCondition=1  SampleTime=-1
  Delay{1,3..5} (4 alike) : Delay  DelayLength=1  InitialCondition=0  UseCircularBuffer=on
  Logical Operator : Logic  Operator=XOR  IconShape=distinctive  AllPortsSameDT=off  OutDataTypeStr=boolean
  Logical Operator1 : Logic  Operator=XOR  IconShape=distinctive  AllPortsSameDT=off  OutDataTypeStr=boolean
  Sample Control Bus Creator : whdlutilities/Sample Control Bus Creator
  StateControl : StateControl  StateControl=Synchronous
  data_out : Outport  SampleTime=0.125
  ctrl_out : Outport  Port=2  SampleTime=0.125
  wires:
  Sample Control Bus Creator/1 -> ctrl_out/1
  Logical Operator1/1 -> C1/1, Logical Operator/2
  Logical Operator/1 -> data_out/1
  [rst] -> C5/3
  [en] -> C5/2
  [en] -> C1/2
  [rst] -> C4/3
  [en] -> C4/2
  [rst] -> C1/3
  [rst] -> C20/3
  [en] -> C20/2
  [rst] -> C19/3
  [en] -> C19/2
  [rst] -> C18/3
  [en] -> C18/2
  [rst] -> C3/3
  [rst] -> C17/3
  [en] -> C17/2
  [rst] -> C23/3
  [en] -> C23/2
  [rst] -> C22/3
  [en] -> C22/2
  [rst] -> C21/3
  [en] -> C21/2
  [rst] -> C13/3
  [en] -> C13/2
  [en] -> C3/2
  [rst] -> C12/3
  [en] -> C12/2
  [rst] -> C11/3
  [en] -> C11/2
  [rst] -> C10/3
  [en] -> C10/2
  [rst] -> C16/3
  [en] -> C16/2
  [rst] -> C15/3
  [en] -> C15/2
  [rst] -> C2/3
  [rst] -> C14/3
  [en] -> C14/2
  [rst] -> C9/3
  [en] -> C9/2
  [rst] -> C8/3
  [en] -> C8/2
  [rst] -> C7/3
  [en] -> C7/2
  [rst] -> C6/3
  [en] -> C6/2
  [en] -> C2/2
  Delay5/1 -> Sample Control Bus Creator/3
  Delay4/1 -> Sample Control Bus Creator/2
  Delay3/1 -> Sample Control Bus Creator/1
  Delay1/1 -> Logical Operator/1
  C9/1 -> C10/1
  C8/1 -> C9/1
  C7/1 -> C8/1
  C6/1 -> C7/1
  C5/1 -> C6/1
  C4/1 -> C5/1
  C3/1 -> C4/1
  C23/1 -> Logical Operator1/1
  C22/1 -> C23/1
  C21/1 -> C22/1
  C20/1 -> C21/1
  C2/1 -> C3/1
  C19/1 -> C20/1
  C18/1 -> C19/1, Logical Operator1/2
  C17/1 -> C18/1
  C16/1 -> C17/1
  C15/1 -> C16/1
  C14/1 -> C15/1
  C13/1 -> C14/1
  C12/1 -> C13/1
  C11/1 -> C12/1
  C10/1 -> C11/1
  C1/1 -> C2/1
  Bus Selector1/3 -> Delay5/1, [en]  "<valid>"
  Bus Selector1/2 -> Delay4/1  "<end>"
  Bus Selector1/1 -> Delay3/1, [rst]  "<start>"
  ctrl_in/1 -> Bus Selector1/1
  data_in/1 -> Delay1/1

== system gm_HDLHeaderFull_vs/header_full/header_fec ==
  data_in : Inport  OutDataTypeStr=boolean  SampleTime=0.125
  ctrl_in : Inport  Port=2  SampleTime=0.125
  Hc_12H_B14 : whdledac/LDPC Encoder  ParityCheckMatrix=Hc_12H  BlockSize=14  SimulateUsing=Code generation
  data_out : Outport  SampleTime=0.125
  ctrl_out : Outport  Port=2  SampleTime=0.125
  next_frame : Outport  Port=3  SampleTime=0.125
  wires:
  Hc_12H_B14/3 -> next_frame/1
  Hc_12H_B14/2 -> ctrl_out/1
  Hc_12H_B14/1 -> data_out/1
  ctrl_in/1 -> Hc_12H_B14/2
  data_in/1 -> Hc_12H_B14/1

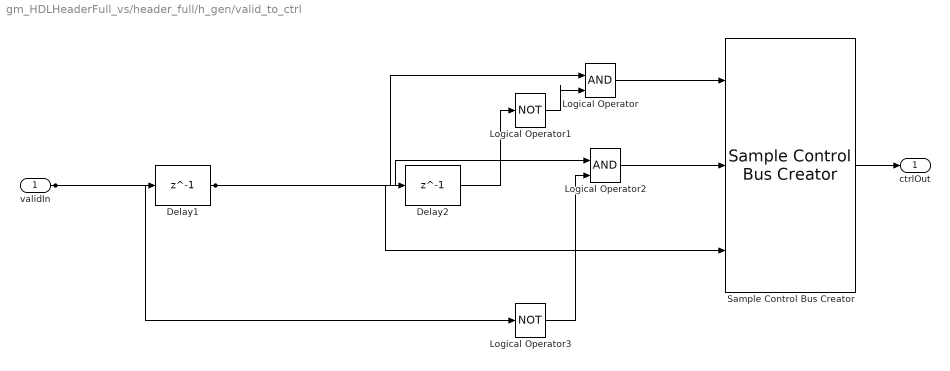
== system gm_HDLHeaderFull_vs/header_full/h_gen/valid_to_ctrl ==
  validIn : Inport  OutDataTypeStr=boolean  SampleTime=0.125
  Delay1 : Delay  DelayLength=1  InitialCondition=0  UseCircularBuffer=on
  Delay2 : Delay  DelayLength=1  InitialCondition=0  UseCircularBuffer=on
  Logical Operator : Logic  IconShape=distinctive  AllPortsSameDT=off  OutDataTypeStr=boolean
  Logical Operator1 : Logic  Operator=NOT  IconShape=distinctive  AllPortsSameDT=off  OutDataTypeStr=boolean
  Logical Operator2 : Logic  IconShape=distinctive  AllPortsSameDT=off  OutDataTypeStr=boolean
  Logical Operator3 : Logic  Operator=NOT  IconShape=distinctive  AllPortsSameDT=off  OutDataTypeStr=boolean
  Sample Control Bus Creator : whdlutilities/Sample Control Bus Creator
  ctrlOut : Outport  SampleTime=0.125
  wires:
  Sample Control Bus Creator/1 -> ctrlOut/1
  Logical Operator3/1 -> Logical Operator2/2
  Logical Operator2/1 -> Sample Control Bus Creator/2
  Logical Operator1/1 -> Logical Operator/2
  Logical Operator/1 -> Sample Control Bus Creator/1
  Delay2/1 -> Logical Operator1/1
  Delay1/1 -> Sample Control Bus Creator/3, Delay2/1, Logical Operator/1, Logical Operator2/1
  validIn/1 -> Delay1/1, Logical Operator3/1
